simulink model "DC_Motor_yt"  (R2021a)
settings: Solver=VariableStepAuto  StartTime=0.0  StopTime=10.0  RelTol=1e-3
libraries: spsDiodeLib x2, spsThyristorLib x2, spsACVoltageSourceLib x1, spsDCMachineLib x1, spsDCVoltageSourceLib x1, spspowerguiLib x1
settings Model: Creator=Sabari Vijayan  LastModifiedBy=Kryptic

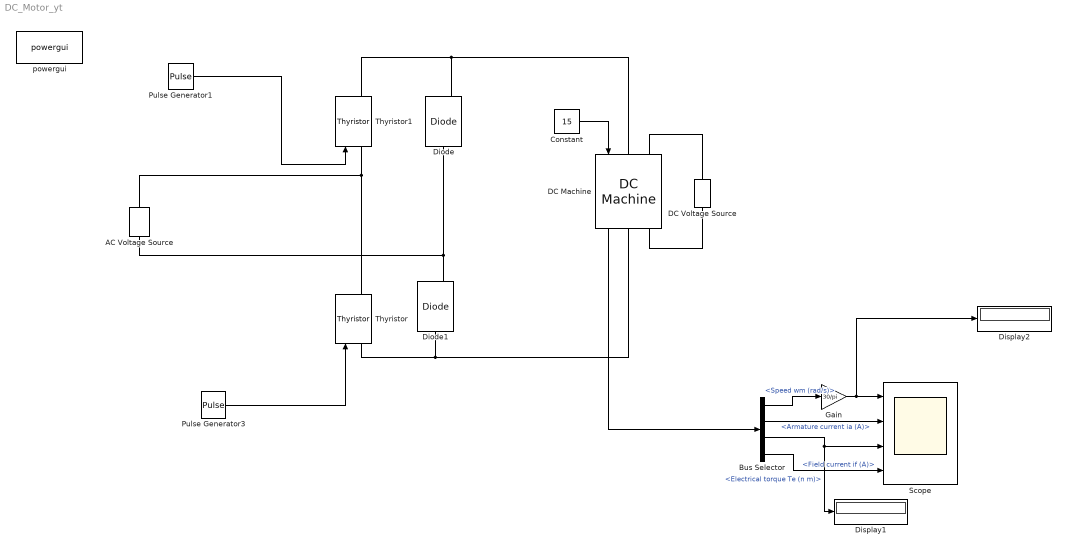
== system DC_Motor_yt ==
  AC Voltage Source : spsACVoltageSourceLib/AC Voltage Source  Amplitude=339  Phase=0  Frequency=50  SampleTime=0  Measurements=None  BusType=swing  Pref=10e3  Qref=0  Qmin=-inf  Qmax=+inf
  Bus Selector : BusSelector  OutputSignals=Speed wm (rad/s),Armature current ia (A),Electrical torque Te (n m),Field current if (A)
  Constant : Constant  Value=15
  DC Machine : spsDCMachineLib/DC Machine  PresetModel=02: 5HP 240V 1750RPM Field:150V  MechanicalLoad=Torque TL  FieldType=Wound  ShowDetailedParameters=on  MeasurementBus=off  RLa=[0.78 0.016]  RLf=[150 112.5]  Laf=1.234  MachineConstant=Torque constant (N.m/A)  Ke=1.8  Kt=1.8  J=0.05  Bm=0.01  Tf=0  w0=1  Ifinit=0.999999997779339  TsPowergui=0  TsBlock=-1
  DC Voltage Source : spsDCVoltageSourceLib/DC Voltage Source  Amplitude=150  Measurements=None
  Diode : spsDiodeLib/Diode  Ron=0.001  Lon=0  Vf=0.8  IC=0  UseSnubber=0  Rs=500  Cs=250e-9  Measurements=on
  Diode1 : spsDiodeLib/Diode  Ron=0.001  Lon=0  Vf=0.8  IC=0  UseSnubber=0  Rs=500  Cs=250e-9  Measurements=on
  Display1 : Display
  Display2 : Display
  Gain : Gain  Gain=30/pi
  Pulse Generator1 : DiscretePulseGenerator  PulseType=Time based  Amplitude=2  Period=1/50  PulseWidth=20  PhaseDelay=0.0015
  Pulse Generator3 : DiscretePulseGenerator  PulseType=Time based  Amplitude=2  Period=1/50  PulseWidth=20  PhaseDelay=0.0115
  Scope : Scope  NumInputPorts=4
  Thyristor : spsThyristorLib/Thyristor  Ron=0.001  Lon=0  Vf=0.8  IC=0  Rs=500  Cs=250e-9  Measurements=on
  Thyristor1 : spsThyristorLib/Thyristor  Ron=0.001  Lon=0  Vf=0.8  IC=0  Rs=500  Cs=250e-9  Measurements=on
  powergui : spspowerguiLib/powergui  Priority=1  SimulationMode=Continuous  SampleTime=50e-6  frequency=60  Iterations=50  frequencyindice=50  Pbase=100e6  ErrMax=1e-4  UnitsV=kV  UnitsW=MW  buscounter=0  FunctionMessages=off  echomessages=off  EnableUseOfTLC=off  CurrentSourceSwitches=off  DisableSnubberDevices=off  DisableRonSwitches=off  DisableVfSwitches=off  DisplayEquations=off  AutomaticDiscreteSolvers=off  SolverType=Tustin/Backward Euler (TBE)  Interpol=off  ExternalGateDelay=off  methode=off  Ts=100  x0status=blocks  SPID=on  SwTol=0  HookPort=off  NonlinearTolerance=1e-4  nMaxIteration=100  ContinueOnMaxIteration=off  RestoreLinks=warning  ResistiveCurrentMeasurement=off  Frange=[0:2:500]  Ylog=off  Xlog=on  ShowGrid=off  save=off  variable=ZData  structure=0  ZoomFFT=off  StartTime=0.0  cycles=1  DisplayStyle=1  fundamental=60  FreqAxis=off  MaxFrequency=1000  frequencyindicesteady=1  RmsSteady=1  display=off
  wires:
  Bus Selector/3 -> Display1/1, Scope/3  "<Electrical torque Te (n m)>"
  Bus Selector/1 -> Gain/1  "<Speed wm (rad/s)>"
  DC Machine/1 -> Bus Selector/1
  Bus Selector/2 -> Scope/2  "<Armature current ia (A)>"
  Constant/1 -> DC Machine/1
  Gain/1 -> Display2/1, Scope/1
  Pulse Generator1/1 -> Thyristor1/1
  Pulse Generator3/1 -> Thyristor/1
  Bus Selector/4 -> Scope/4  "<Field current if (A)>"
  connections:
  DC Machine/RConn1 -- Thyristor/LConn1 -- Diode1/LConn1
  Thyristor1/LConn1 -- AC Voltage Source/RConn1 -- Thyristor/RConn1
  AC Voltage Source/LConn1 -- Diode1/RConn1 -- Diode/LConn1
  Thyristor1/RConn1 -- DC Machine/LConn1 -- Diode/RConn1
  DC Machine/RConn2 -- DC Voltage Source/LConn1
  DC Machine/LConn2 -- DC Voltage Source/RConn1
